simulink model "svpwm"  (R2020a)
settings: Solver=VariableStepAuto  StartTime=0.0  StopTime=.1  RelTol=1e-3
libraries: simulink x13, powerlib_meascontrol x1, powerlib x1
settings Model: Creator=hp  LastModifiedBy=hp

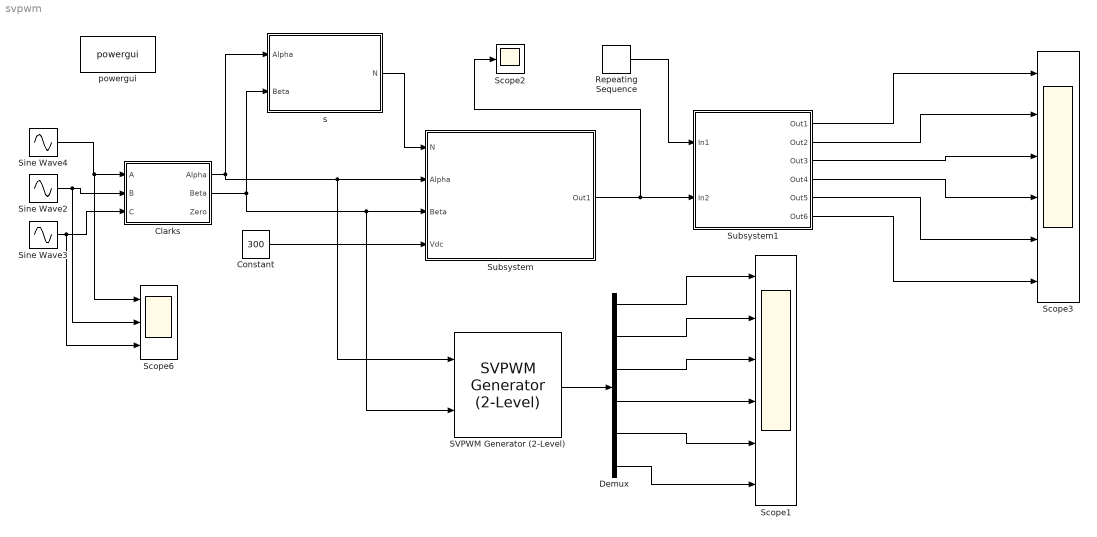
== system svpwm ==
  Clarks : Subsystem
  Constant : Constant  Value=300
  Demux : Demux  Outputs=6
  Repeating Sequence : simulink/Sources/Repeating Sequence  rep_seq_t=[0 .0005 .001]  rep_seq_y=[0 1 0]
  SVPWM Generator (2-Level) : powerlib_meascontrol/Pulse & Signal Generators/SVPWM Generator (2-Level)  InputType=alpha-beta components  SwitchingPattern=Pattern #1  Fc=1000  ParUref=[0.8 -30 50]  Ts=0
      settings: SourceProductBaseCode=PS
  Scope1 : Scope  NumInputPorts=6
  Scope2 : Scope
  Scope3 : Scope  NumInputPorts=6
  Scope6 : Scope  NumInputPorts=3
  Sine Wave2 : Sin  Amplitude=100  Frequency=2*pi*50  Phase=(2*pi)/3  SampleTime=5e-6
  Sine Wave3 : Sin  Amplitude=100  Frequency=2*pi*50  Phase=(4*pi)/3  SampleTime=5e-6
  Sine Wave4 : Sin  Amplitude=100  Frequency=2*pi*50  SampleTime=5e-6
  Subsystem : Subsystem
  Subsystem1 : Subsystem
  powergui : powerlib/powergui  Priority=1  SimulationMode=Discrete  SampleTime=50e-6  frequency=60  Iterations=50  frequencyindice=60  Pbase=100e6  ErrMax=1e-4  UnitsV=kV  UnitsW=MW  buscounter=0  FunctionMessages=off  echomessages=off  EnableUseOfTLC=off  CurrentSourceSwitches=off  DisableSnubberDevices=off  DisableRonSwitches=off  DisableVfSwitches=off  DisplayEquations=off  AutomaticDiscreteSolvers=off  SolverType=Tustin/Backward Euler (TBE)  Interpol=off  ExternalGateDelay=off  methode=off  Ts=100  x0status=blocks  SPID=on  SwTol=0  HookPort=off  NonlinearTolerance=1e-4  nMaxIteration=100  ContinueOnMaxIteration=off  RestoreLinks=warning  ResistiveCurrentMeasurement=off  Frange=[0:2:500]  Ylog=off  Xlog=on  ShowGrid=off  save=off  variable=ZData  structure=0  ZoomFFT=off  StartTime=0.0  cycles=1  DisplayStyle=1  fundamental=60  FreqAxis=off  MaxFrequency=1000  frequencyindicesteady=1  RmsSteady=1  display=off
  s : Subsystem
  wires:
  Clarks/1(Alpha) -> SVPWM Generator (2-Level)/1, Subsystem/2(Alpha), s/1(Alpha)
  Sine Wave2/1 -> Scope6/2, Clarks/2(B)
  Sine Wave3/1 -> Scope6/3, Clarks/3(C)
  Sine Wave4/1 -> Scope6/1, Clarks/1(A)
  Clarks/2(Beta) -> SVPWM Generator (2-Level)/2, Subsystem/3(Beta), s/2(Beta)
  Subsystem/1(Out1) -> Subsystem1/2(In2), Scope2/1
  s/1(N) -> Subsystem/1(N)
  Constant/1 -> Subsystem/4(Vdc)
  Repeating Sequence/1 -> Subsystem1/1(In1)
  Subsystem1/1(Out1) -> Scope3/1
  Subsystem1/2(Out2) -> Scope3/2
  Subsystem1/3(Out3) -> Scope3/3
  Subsystem1/4(Out4) -> Scope3/4
  Subsystem1/5(Out5) -> Scope3/5
  Subsystem1/6(Out6) -> Scope3/6
  SVPWM Generator (2-Level)/1 -> Demux/1
  Demux/1 -> Scope1/1
  Demux/2 -> Scope1/2
  Demux/3 -> Scope1/3
  Demux/4 -> Scope1/4
  Demux/5 -> Scope1/5
  Demux/6 -> Scope1/6

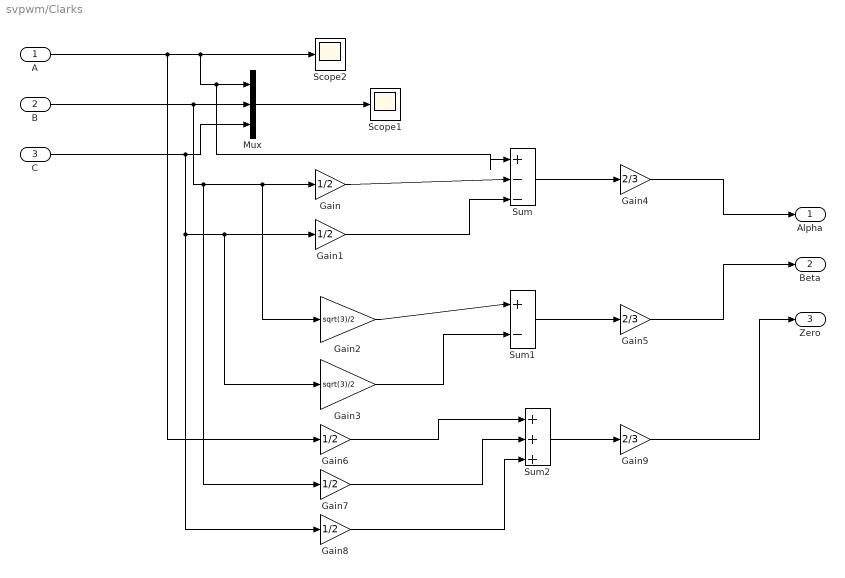
== system svpwm/Clarks ==
  A : Inport
  B : Inport  Port=2
  C : Inport  Port=3
  Gain{,1,6..8} (5 alike) : Gain  Gain=1/2
  Gain2 : Gain  Gain=sqrt(3)/2
  Gain3 : Gain  Gain=sqrt(3)/2
  Gain4 : Gain  Gain=2/3
  Gain5 : Gain  Gain=2/3
  Gain9 : Gain  Gain=2/3
  Mux : Mux  Inputs=3
  Scope1 : Scope
  Scope2 : Scope
  Sum : Sum  Inputs=|+--
  Sum1 : Sum  Inputs=|+-
  Sum2 : Sum  Inputs=|+++
  Alpha : Outport
  Beta : Outport  Port=2
  Zero : Outport  Port=3
  wires:
  A/1 -> Gain6/1, Sum/1, Mux/1, Scope2/1
  Gain8/1 -> Sum2/3
  Mux/1 -> Scope1/1
  Gain/1 -> Sum/2
  Gain4/1 -> Alpha/1
  Gain3/1 -> Sum1/2
  B/1 -> Gain7/1, Gain2/1, Gain/1, Mux/2
  C/1 -> Gain8/1, Gain3/1, Gain1/1, Mux/3
  Sum1/1 -> Gain5/1
  Gain7/1 -> Sum2/2
  Gain2/1 -> Sum1/1
  Sum2/1 -> Gain9/1
  Gain6/1 -> Sum2/1
  Sum/1 -> Gain4/1
  Gain1/1 -> Sum/3
  Gain5/1 -> Beta/1
  Gain9/1 -> Zero/1

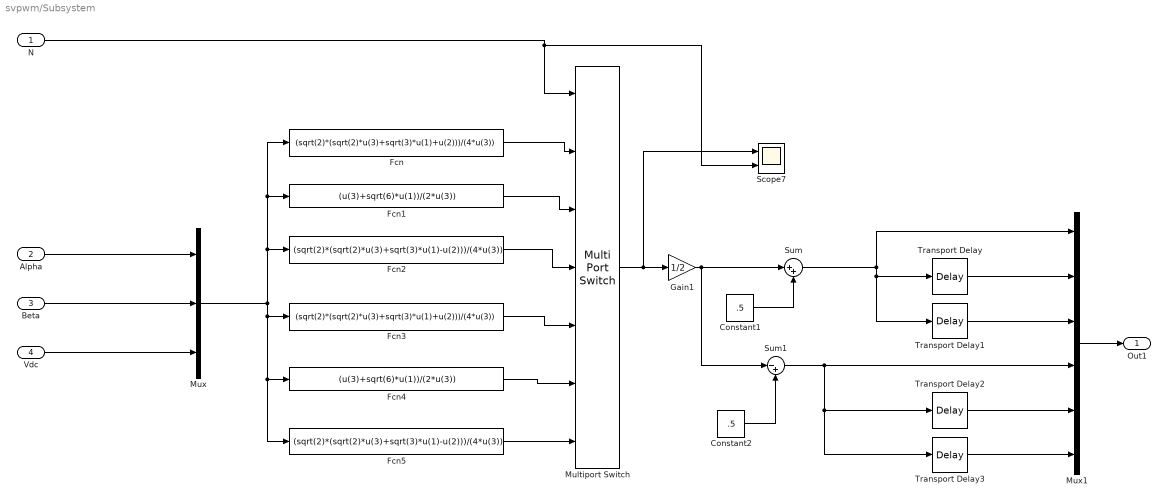
== system svpwm/Subsystem ==
  N : Inport
  Alpha : Inport  Port=2
  Beta : Inport  Port=3
  Vdc : Inport  Port=4
  Constant1 : Constant  Value=.5
  Constant2 : Constant  Value=.5
  Fcn : Fcn  Expr=(sqrt(2)*(sqrt(2)*u(3)+sqrt(3)*u(1)+u(2)))/(4*u(3))
  Fcn1 : Fcn  Expr=(u(3)+sqrt(6)*u(1))/(2*u(3))
  Fcn2 : Fcn  Expr=(sqrt(2)*(sqrt(2)*u(3)+sqrt(3)*u(1)-u(2)))/(4*u(3))
  Fcn3 : Fcn  Expr=(sqrt(2)*(sqrt(2)*u(3)+sqrt(3)*u(1)+u(2)))/(4*u(3))
  Fcn4 : Fcn  Expr=(u(3)+sqrt(6)*u(1))/(2*u(3))
  Fcn5 : Fcn  Expr=(sqrt(2)*(sqrt(2)*u(3)+sqrt(3)*u(1)-u(2)))/(4*u(3))
  Gain1 : Gain  Gain=1/2
  Multiport Switch : MultiPortSwitch  Inputs=6
  Mux : Mux  Inputs=3
  Mux1 : Mux  Inputs=6
  Scope7 : Scope  NumInputPorts=2
  Sum : Sum  Inputs=|++
  Sum1 : Sum  Inputs=|-+
  Transport Delay : TransportDelay  DelayTime=.02/3  InitialOutput=.75
  Transport Delay1 : TransportDelay  DelayTime=2*(.02/3)  InitialOutput=.75
  Transport Delay2 : TransportDelay  DelayTime=.02/3  InitialOutput=.25
  Transport Delay3 : TransportDelay  DelayTime=2*(.02/3)  InitialOutput=.25
  Out1 : Outport
  wires:
  N/1 -> Multiport Switch/1, Scope7/2
  Gain1/1 -> Sum1/1, Sum/1
  Transport Delay3/1 -> Mux1/6
  Sum1/1 -> Mux1/4, Transport Delay3/1, Transport Delay2/1
  Constant1/1 -> Sum/2
  Fcn/1 -> Multiport Switch/2
  Multiport Switch/1 -> Scope7/1, Gain1/1
  Fcn3/1 -> Multiport Switch/5
  Sum/1 -> Mux1/1, Transport Delay1/1, Transport Delay/1
  Mux/1 -> Fcn5/1, Fcn4/1, Fcn3/1, Fcn2/1, Fcn1/1, Fcn/1
  Fcn2/1 -> Multiport Switch/4
  Beta/1 -> Mux/2
  Fcn1/1 -> Multiport Switch/3
  Transport Delay1/1 -> Mux1/3
  Fcn5/1 -> Multiport Switch/7
  Transport Delay/1 -> Mux1/2
  Constant2/1 -> Sum1/2
  Alpha/1 -> Mux/1
  Fcn4/1 -> Multiport Switch/6
  Transport Delay2/1 -> Mux1/5
  Mux1/1 -> Out1/1
  Vdc/1 -> Mux/3

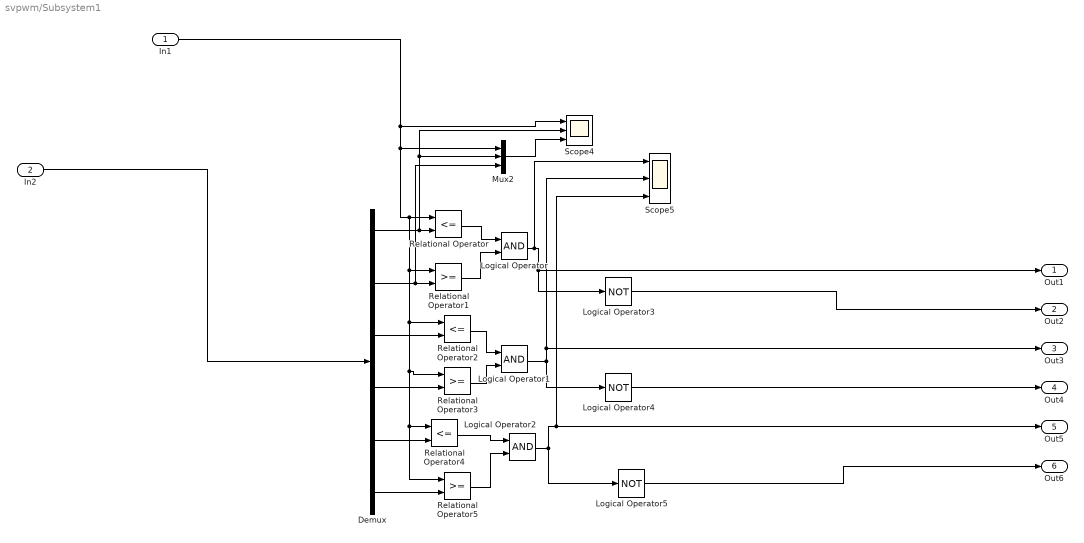
== system svpwm/Subsystem1 ==
  In1 : Inport
  In2 : Inport  Port=2
  Demux : Demux  Outputs=6
  Logical Operator : Logic  AllPortsSameDT=off  OutDataTypeStr=boolean
  Logical Operator1 : Logic  AllPortsSameDT=off  OutDataTypeStr=boolean
  Logical Operator2 : Logic  AllPortsSameDT=off  OutDataTypeStr=boolean
  Logical Operator3 : Logic  Operator=NOT  AllPortsSameDT=off  OutDataTypeStr=boolean
  Logical Operator4 : Logic  Operator=NOT  AllPortsSameDT=off  OutDataTypeStr=boolean
  Logical Operator5 : Logic  Operator=NOT  AllPortsSameDT=off  OutDataTypeStr=boolean
  Mux2 : Mux  Inputs=3
  Relational Operator : RelationalOperator  Operator=<=  OutDataTypeStr=boolean  RndMeth=Simplest
  Relational Operator1 : RelationalOperator  OutDataTypeStr=boolean  RndMeth=Simplest
  Relational Operator2 : RelationalOperator  Operator=<=  OutDataTypeStr=boolean  RndMeth=Simplest
  Relational Operator3 : RelationalOperator  OutDataTypeStr=boolean  RndMeth=Simplest
  Relational Operator4 : RelationalOperator  Operator=<=  OutDataTypeStr=boolean  RndMeth=Simplest
  Relational Operator5 : RelationalOperator  OutDataTypeStr=boolean  RndMeth=Simplest
  Scope4 : Scope  NumInputPorts=3
  Scope5 : Scope  NumInputPorts=3
  Out1 : Outport
  Out2 : Outport  Port=2
  Out3 : Outport  Port=3
  Out4 : Outport  Port=4
  Out5 : Outport  Port=5
  Out6 : Outport  Port=6
  wires:
  Demux/4 -> Relational Operator3/2
  Demux/1 -> Mux2/2, Scope4/2, Relational Operator/2
  In1/1 -> Scope4/1, Relational Operator1/1, Relational Operator3/1, Relational Operator5/1, Relational Operator4/1, Relational Operator2/1, Relational Operator/1, Mux2/1
  Demux/3 -> Relational Operator2/2
  Demux/6 -> Relational Operator5/2
  Demux/2 -> Mux2/3, Relational Operator1/2
  Logical Operator3/1 -> Out2/1
  Relational Operator1/1 -> Logical Operator/2
  Relational Operator/1 -> Logical Operator/1
  Logical Operator1/1 -> Logical Operator4/1, Out3/1, Scope5/2
  In2/1 -> Demux/1
  Relational Operator2/1 -> Logical Operator1/1
  Logical Operator/1 -> Scope5/1, Out1/1, Logical Operator3/1
  Demux/5 -> Relational Operator4/2
  Relational Operator4/1 -> Logical Operator2/1
  Relational Operator3/1 -> Logical Operator1/2
  Relational Operator5/1 -> Logical Operator2/2
  Logical Operator2/1 -> Logical Operator5/1, Out5/1, Scope5/3
  Mux2/1 -> Scope4/3
  Logical Operator4/1 -> Out4/1
  Logical Operator5/1 -> Out6/1

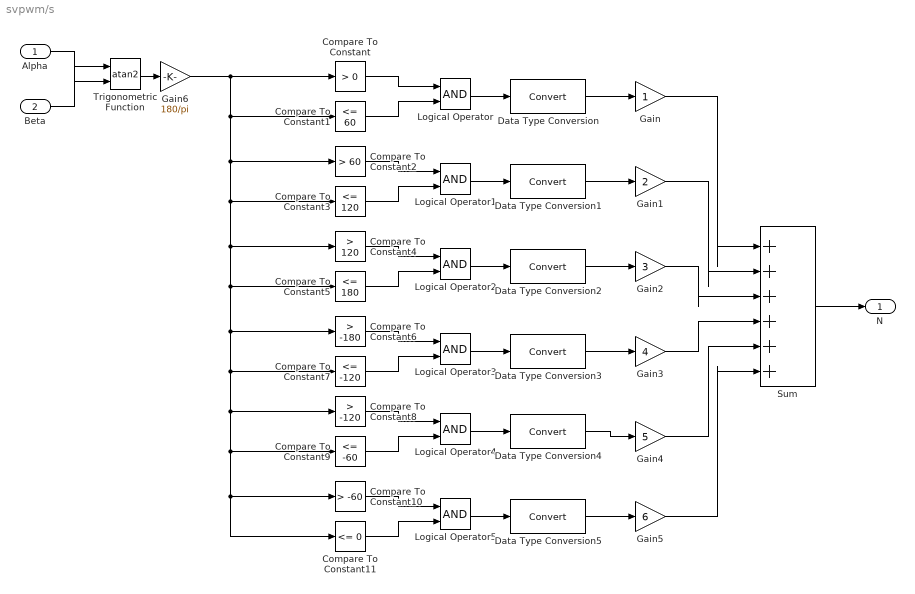
== system svpwm/s ==
  Alpha : Inport
  Beta : Inport  Port=2
  Compare To Constant : simulink/Logic and Bit Operations/Compare To Constant  relop=>  const=0  OutDataTypeStr=boolean
  Compare To Constant1 : simulink/Logic and Bit Operations/Compare To Constant  relop=<=  const=60  OutDataTypeStr=boolean
  Compare To Constant10 : simulink/Logic and Bit Operations/Compare To Constant  relop=>  const=-60  OutDataTypeStr=boolean
  Compare To Constant11 : simulink/Logic and Bit Operations/Compare To Constant  relop=<=  const=0  OutDataTypeStr=boolean
  Compare To Constant2 : simulink/Logic and Bit Operations/Compare To Constant  relop=>  const=60  OutDataTypeStr=boolean
  Compare To Constant3 : simulink/Logic and Bit Operations/Compare To Constant  relop=<=  const=120  OutDataTypeStr=boolean
  Compare To Constant4 : simulink/Logic and Bit Operations/Compare To Constant  relop=>  const=120  OutDataTypeStr=boolean
  Compare To Constant5 : simulink/Logic and Bit Operations/Compare To Constant  relop=<=  const=180  OutDataTypeStr=boolean
  Compare To Constant6 : simulink/Logic and Bit Operations/Compare To Constant  relop=>  const=-180  OutDataTypeStr=boolean
  Compare To Constant7 : simulink/Logic and Bit Operations/Compare To Constant  relop=<=  const=-120  OutDataTypeStr=boolean
  Compare To Constant8 : simulink/Logic and Bit Operations/Compare To Constant  relop=>  const=-120  OutDataTypeStr=boolean
  Compare To Constant9 : simulink/Logic and Bit Operations/Compare To Constant  relop=<=  const=-60  OutDataTypeStr=boolean
  Data Type Conversion{,1..5} (6 alike) : DataTypeConversion
  Gain : Gain
  Gain1 : Gain  Gain=2
  Gain2 : Gain  Gain=3
  Gain3 : Gain  Gain=4
  Gain4 : Gain  Gain=5
  Gain5 : Gain  Gain=6
  Gain6 : Gain  Gain=180/pi
  Logical Operator{,1..5} (6 alike) : Logic  AllPortsSameDT=off  OutDataTypeStr=boolean
  Sum : Sum  Inputs=|++++++
  Trigonometric Function : Trigonometry  Operator=atan2
  N : Outport
  wires:
  Beta/1 -> Trigonometric Function/1
  Alpha/1 -> Trigonometric Function/2
  Compare To Constant/1 -> Logical Operator/1
  Compare To Constant1/1 -> Logical Operator/2
  Logical Operator/1 -> Data Type Conversion/1
  Logical Operator1/1 -> Data Type Conversion1/1
  Compare To Constant3/1 -> Logical Operator1/2
  Compare To Constant2/1 -> Logical Operator1/1
  Compare To Constant4/1 -> Logical Operator2/1
  Compare To Constant5/1 -> Logical Operator2/2
  Logical Operator2/1 -> Data Type Conversion2/1
  Logical Operator3/1 -> Data Type Conversion3/1
  Compare To Constant7/1 -> Logical Operator3/2
  Compare To Constant6/1 -> Logical Operator3/1
  Compare To Constant8/1 -> Logical Operator4/1
  Compare To Constant9/1 -> Logical Operator4/2
  Logical Operator4/1 -> Data Type Conversion4/1
  Logical Operator5/1 -> Data Type Conversion5/1
  Compare To Constant11/1 -> Logical Operator5/2
  Compare To Constant10/1 -> Logical Operator5/1
  Trigonometric Function/1 -> Gain6/1
  Data Type Conversion/1 -> Gain/1
  Data Type Conversion1/1 -> Gain1/1
  Data Type Conversion2/1 -> Gain2/1
  Data Type Conversion3/1 -> Gain3/1
  Data Type Conversion4/1 -> Gain4/1
  Data Type Conversion5/1 -> Gain5/1
  Gain/1 -> Sum/1
  Gain1/1 -> Sum/2
  Gain2/1 -> Sum/3
  Gain3/1 -> Sum/4
  Gain4/1 -> Sum/5
  Gain5/1 -> Sum/6
  Sum/1 -> N/1
  Gain6/1 -> Compare To Constant5/1, Compare To Constant6/1, Compare To Constant10/1, Compare To Constant11/1, Compare To Constant9/1, Compare To Constant8/1, Compare To Constant7/1, Compare To Constant4/1, Compare To Constant3/1, Compare To Constant2/1, Compare To Constant1/1, Compare To Constant/1
